simulink model "Sim_model_nosupervisor"  (Simulink 8.4)
settings: Solver=ode45  StartTime=0.0  StopTime=110  RelTol=1e-3
libraries: simulink x1
CloseFcn:
  | rtwprivate ssgensfun ModelCloseRequest nlgentpl
settings Model: Creator=lbusoniu  LastModifiedBy=Nikhil  ExtModeAutoUpdateStatusClock=off  BufferReuse=off
settings DataIOCC: SaveOutput=off  SaveTime=off  SignalLoggingName=sigsOut
settings OptimizationCC: OptimizeBlockIOStorage=off  BufferReuse=off  GlobalBufferReuse=off  ExpressionFolding=off  ExpressionDepthLimit=128  LocalBlockOutputs=off  InitFltsAndDblsToZero=on
settings DebuggingCC: SaveWithParameterizedLinksMsg=none  SignalResolutionControl=TryResolveAllWithWarning  SolverPrmCheckMsg=none  MultiTaskDSMMsg=warning  MultiTaskCondExecSysMsg=none  StateNameClashWarn=none
settings HardwareCC: TargetUnknown=on
settings RTWCC: IncludeERTFirstTime=on
settings GRTTargetCC: TargetFcnLib=ansi_tfl_tmw.mat

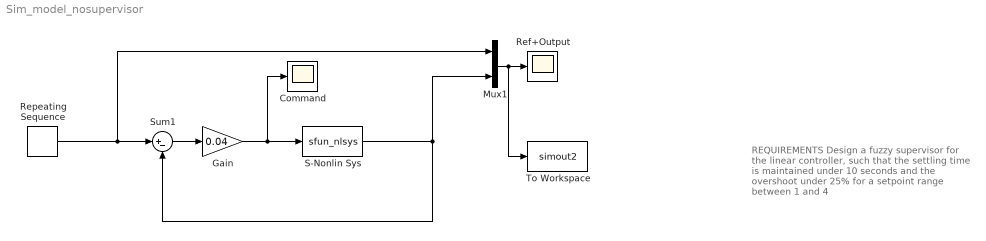
== system Sim_model_nosupervisor ==
  note: REQUIREMENTS
      | Design a fuzzy supervisor for the linear controller, such that
      | the settling time is maintained under 10 seconds and the overshoot under 25%
      | for a setpoint range between 1 and 4
  Command : Scope
      settings: TimeRange=120  YMin=-0.05  YMax=0.15  SaveName=u
  Gain : Gain  Gain=0.04
  Mux1 : Mux  Inputs=2
  Ref+Output : Scope
      settings: TimeRange=120  YMin=0  SaveName=u2
  Repeating Sequence : simulink/Sources/Repeating Sequence  rep_seq_t=[0 15 15.5 30 30.5 45 45.5 60 60.5 75 75.5 90 91.5 111]  rep_seq_y=[1 1 .5 .5 2 2 1.5 1.5 3 3 2.5 2.5 4 4]
  S-Nonlin Sys : S-Function  FunctionName=sfun_nlsys  EnableBusSupport=off
  Sum1 : Sum  Inputs=|+-  SaturateOnIntegerOverflow=on
  To Workspace : ToWorkspace  VariableName=simout2  SaveFormat=Timeseries  SampleTime=-1
  wires:
  Sum1/1 -> Gain/1
  S-Nonlin Sys/1 -> Sum1/2, Mux1/2
  Gain/1 -> S-Nonlin Sys/1, Command/1
  Mux1/1 -> To Workspace/1, Ref+Output/1
  Repeating Sequence/1 -> Sum1/1, Mux1/1
